simulink model "PassiveQuarterCar"  (R2025b)
settings: Solver=VariableStepAuto  StartTime=0.0  StopTime=10.0  RelTol=1e-3
values from neighbouring files (symbols this model uses):
  cs = 1500    [RegenVariables.mat]
  ks = 18000    [RegenVariables.mat]
  kt = 200000    [RegenVariables.mat]
  ms = 320    [RegenVariables.mat]
  mu = 45    [RegenVariables.mat]
settings Model: Creator=khalidwaleed  LastModifiedBy=khalidwaleed

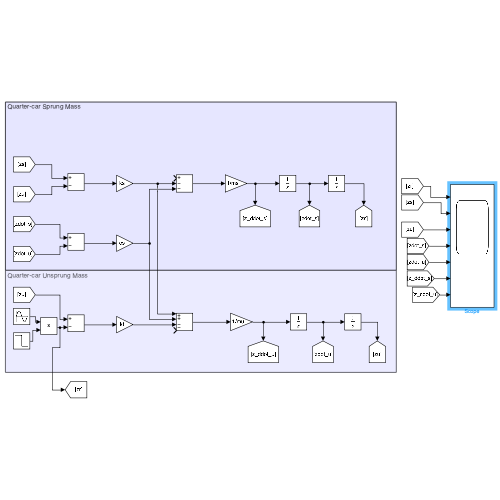
[thumbnail: Simulink's stored preview of the top-level diagram]
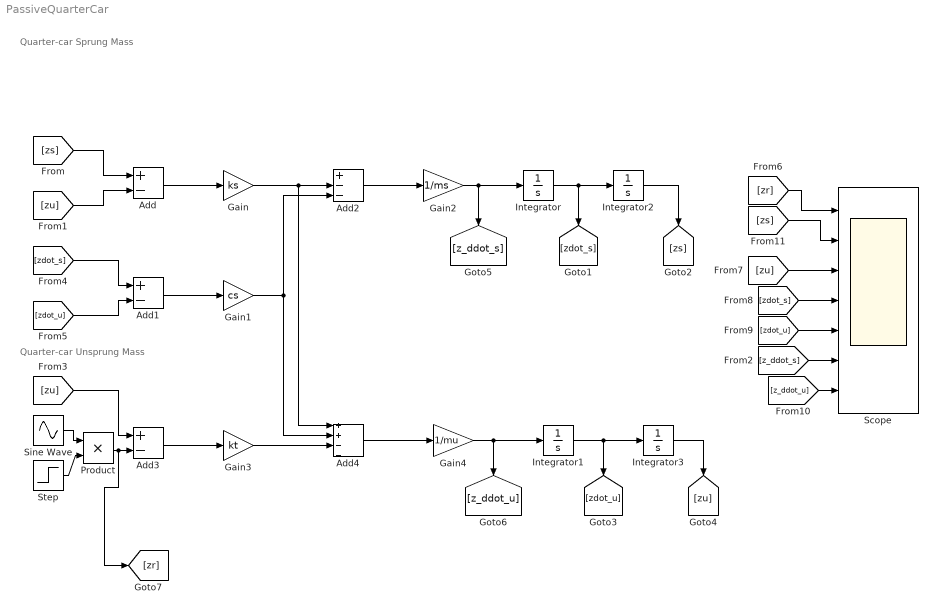
== system PassiveQuarterCar ==
  note: Quarter-car Sprung Mass
  note: Quarter-car Unsprung Mass
  Add : Sum  Inputs=+-
  Add1 : Sum  Inputs=+-
  Add2 : Sum  Inputs=+--
  Add3 : Sum  Inputs=+-
  Add4 : Sum  Inputs=++--
  Gain : Gain  Gain=ks
  Gain1 : Gain  Gain=cs
  Gain2 : Gain  Gain=1/ms
  Gain3 : Gain  Gain=kt
  Gain4 : Gain  Gain=1/mu
  Integrator{,1..3} (4 alike) : Integrator
  Product : Product
  Scope : Scope  NumInputPorts=7
      settings: ActiveDisplayYMinimum=-0.018747687622342017  ActiveDisplayYMaximum=0.16872918860107819
  Sine Wave : Sin  Amplitude=0.15  Frequency=2*pi  SampleTime=0
  Step : Step  Time=0.48  Before=1  After=0  SampleTime=0
  wires:
  Add4/1 -> Gain4/1
  Add2/1 -> Gain2/1
  Integrator/1 -> Integrator2/1, [zdot_s]
  Gain3/1 -> Add4/3
  Add1/1 -> Gain1/1
  Gain1/1 -> Add4/2, Add2/3
  Add/1 -> Gain/1
  [zs] -> Add/1
  Integrator1/1 -> Integrator3/1, [zdot_u]
  Gain4/1 -> Integrator1/1, [z_ddot_u]
  [zu] -> Add3/1
  [zu] -> Add/2
  Step/1 -> Product/2
  [zdot_s] -> Add1/1
  [zdot_u] -> Add1/2
  Integrator3/1 -> [zu]
  Gain/1 -> Add4/1, Add2/2
  Add3/1 -> Gain3/1
  Integrator2/1 -> [zs]
  Gain2/1 -> Integrator/1, [z_ddot_s]
  Sine Wave/1 -> Product/1
  Product/1 -> [zr], Add3/2
  [z_ddot_s] -> Scope/6
  [zs] -> Scope/2
  [zr] -> Scope/1
  [zu] -> Scope/3
  [zdot_s] -> Scope/4
  [zdot_u] -> Scope/5
  [z_ddot_u] -> Scope/7
